simulink model "DCModel"  (Simulink 7.7)
settings: Solver=ode45  StartTime=0.0  StopTime=0.1  RelTol=1e-3
undefined symbols (not defined in the file): B, J, K1, Kc, L, R
settings Model: Creator=Daniel  LastModifiedBy=Daniel

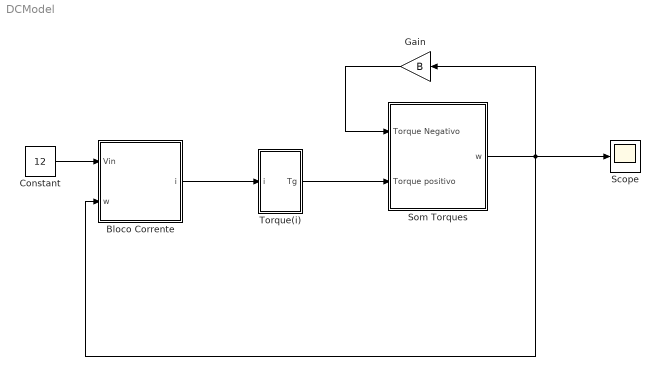
== system DCModel ==
  Bloco Corrente : Subsystem
  Constant : Constant  Value=12
  Gain : Gain  Gain=B
  Scope : Scope
  Som Torques : Subsystem
  Torque(i) : Subsystem
  wires:
  Bloco Corrente/1(i) -> Torque(i)/1(i)
  Torque(i)/1(Tg) -> Som Torques/2(Torque positivo)
  Constant/1 -> Bloco Corrente/1(Vin)
  Som Torques/1(w) -> Bloco Corrente/2(w), Scope/1, Gain/1
  Gain/1 -> Som Torques/1(Torque Negativo)

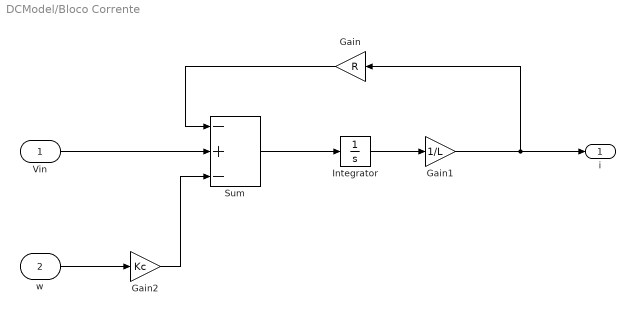
== system DCModel/Bloco Corrente ==
  Vin : Inport
  w : Inport  Port=2
  Gain : Gain  Gain=R
  Gain1 : Gain  Gain=1/L
  Gain2 : Gain  Gain=Kc
  Integrator : Integrator
  Sum : Sum  Inputs=-+-
  i : Outport
  wires:
  Sum/1 -> Integrator/1
  Integrator/1 -> Gain1/1
  w/1 -> Gain2/1
  Gain1/1 -> i/1, Gain/1
  Gain2/1 -> Sum/3
  Vin/1 -> Sum/2
  Gain/1 -> Sum/1

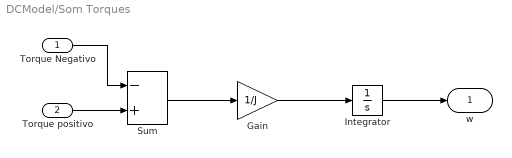
== system DCModel/Som Torques ==
  Torque Negativo : Inport
  Torque positivo : Inport  Port=2
  Gain : Gain  Gain=1/J
  Integrator : Integrator
  Sum : Sum  Inputs=-+
  w : Outport
  wires:
  Torque Negativo/1 -> Sum/1
  Torque positivo/1 -> Sum/2
  Sum/1 -> Gain/1
  Gain/1 -> Integrator/1
  Integrator/1 -> w/1

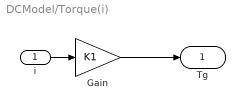
== system DCModel/Torque(i) ==
  i : Inport
  Gain : Gain  Gain=K1
  Tg : Outport
  wires:
  Gain/1 -> Tg/1
  i/1 -> Gain/1
